simulink model "untitled"  (R2018a)
settings: Solver=VariableStepAuto  StartTime=0.0  StopTime=10.0  RelTol=1e-3
settings Model: Creator=Administrator  LastModifiedBy=Administrator

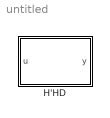
== system untitled ==
  H'HD : MATLAB Function  TreatAsAtomicUnit=on

== matlab function untitled/H'HD ==
  data: u input; y output
function y = fcn(u)

k=0:

y = u;
